simulink model "PathManager"  (R2018a)
settings: Solver=VariableStepAuto  StartTime=0.0  StopTime=10.0  RelTol=1e-3
undefined symbols (not defined in the file): check, SkywalkerX8
settings Model: Creator=David  LastModifiedBy=David

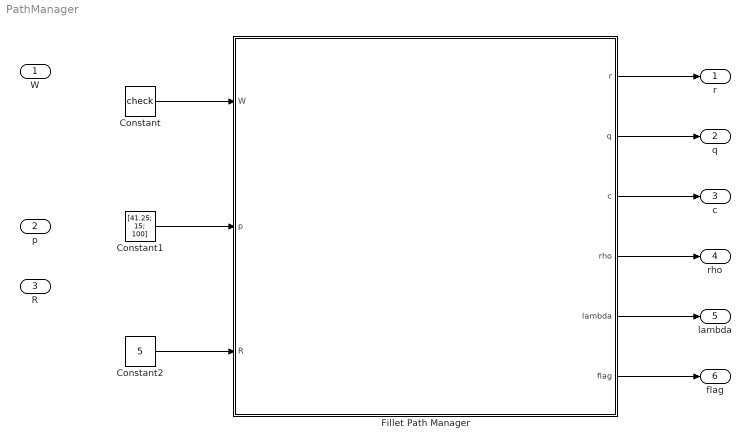
== system PathManager ==
  W : Inport
  p : Inport  Port=2
  R : Inport  Port=3
  Constant : Constant  Value=check
  Constant1 : Constant  Value=[41.25; 15; 100]
  Constant2 : Constant  Value=5
  Fillet Path Manager : Subsystem  mask{SampleTime=SkywalkerX8.GuidanceAndNavigation.SampleTime}
      mask prompts: SampleTime "Sample time (s)"
      mask DialogControl DescGroupVar Prompt: Path Manager
      mask DialogControl DescTextVar Prompt: Path manager which switches between straight line and orbit following using a fillet between waypoint transitions
      mask Display:
      | image('path_planning.png')
      | 
      | port_label('input', 1, '\bf{W} (m)', 'texMode', 'On')
      | port_label('input', 2, '\bf{p} (m)', 'texMode', 'On')
      | port_label('input', 3, 'R (m)', 'texMode', 'On')
      | 
      | port_label('output', 1, '\bf{r} (m)', 'texMode', 'On')
      | port_label('output', 2, '\bf{q} (m)', 'texMode', 'On')
      | port_label('output', 3, '\bf{c} (m)', 'texMode', 'On')
      | port_label('output', 4, '\rho (m)', 'texMode', 'On')
      | port_label('output', 5, '\lambda (m)', 'texMode', 'On')
      | port_label('output', 6, 'Flag (Unitless)', 'texMode', 'On')
  r : Outport
  q : Outport  Port=2
  c : Outport  Port=3
  rho : Outport  Port=4
  lambda : Outport  Port=5
  flag : Outport  Port=6
  wires:
  Constant/1 -> Fillet Path Manager/1(W)
  Constant1/1 -> Fillet Path Manager/2(p)
  Fillet Path Manager/1(r) -> r/1
  Fillet Path Manager/2(q) -> q/1
  Fillet Path Manager/3(c) -> c/1
  Fillet Path Manager/4(rho) -> rho/1
  Fillet Path Manager/5(lambda) -> lambda/1
  Fillet Path Manager/6(flag) -> flag/1
  Constant2/1 -> Fillet Path Manager/3(R)

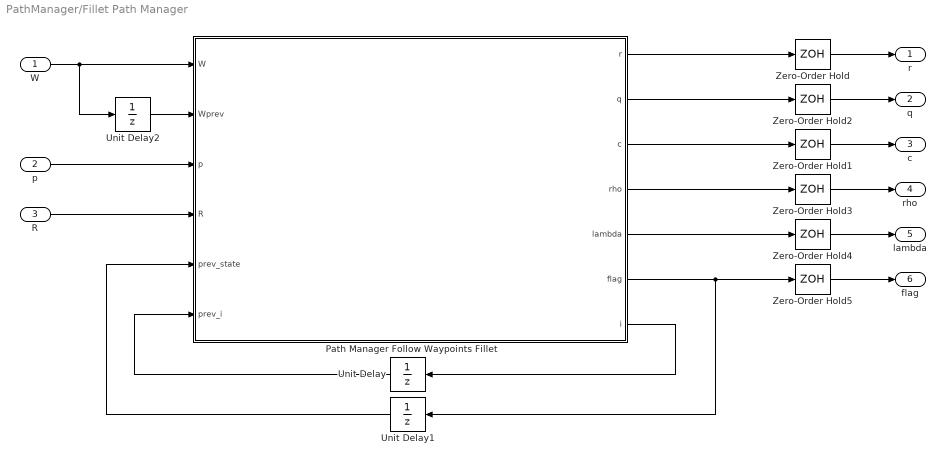
== system PathManager/Fillet Path Manager ==
  W : Inport
  p : Inport  Port=2
  R : Inport  Port=3
  Path Manager Follow Waypoints Fillet : MATLAB Function  TreatAsAtomicUnit=on
  Unit Delay : UnitDelay  InitialCondition=2  SampleTime=SampleTime
  Unit Delay1 : UnitDelay  InitialCondition=1  SampleTime=SampleTime
  Unit Delay2 : UnitDelay  SampleTime=SampleTime
  Zero-Order Hold{,1..5} (6 alike) : ZeroOrderHold  SampleTime=SampleTime
  r : Outport
  q : Outport  Port=2
  c : Outport  Port=3
  rho : Outport  Port=4
  lambda : Outport  Port=5
  flag : Outport  Port=6
  wires:
  Path Manager Follow Waypoints Fillet/2(q) -> Zero-Order Hold2/1
  Path Manager Follow Waypoints Fillet/6(flag) -> Zero-Order Hold5/1, Unit Delay1/1
  W/1 -> Unit Delay2/1, Path Manager Follow Waypoints Fillet/1(W)
  Unit Delay/1 -> Path Manager Follow Waypoints Fillet/6(prev_i)
  Path Manager Follow Waypoints Fillet/7(i) -> Unit Delay/1
  Path Manager Follow Waypoints Fillet/3(c) -> Zero-Order Hold1/1
  p/1 -> Path Manager Follow Waypoints Fillet/3(p)
  Path Manager Follow Waypoints Fillet/4(rho) -> Zero-Order Hold3/1
  Unit Delay2/1 -> Path Manager Follow Waypoints Fillet/2(Wprev)
  Path Manager Follow Waypoints Fillet/1(r) -> Zero-Order Hold/1
  Unit Delay1/1 -> Path Manager Follow Waypoints Fillet/5(prev_state)
  R/1 -> Path Manager Follow Waypoints Fillet/4(R)
  Zero-Order Hold/1 -> r/1
  Zero-Order Hold1/1 -> c/1
  Zero-Order Hold2/1 -> q/1
  Zero-Order Hold3/1 -> rho/1
  Zero-Order Hold4/1 -> lambda/1
  Zero-Order Hold5/1 -> flag/1
  Path Manager Follow Waypoints Fillet/5(lambda) -> Zero-Order Hold4/1

== matlab function PathManager/Fillet Path Manager/Path Manager Follow Waypoints Fillet ==
  data: r output size=3, 1; q output size=3, 1; c output size=3, 1; rho output size=1; lambda output size=1; W input; flag output size=1; Wprev input; p input size=3, 1; R input; prev_state input; prev_i input; i output size=1
function [r, q, c, rho, lambda, flag, i] = fcn(W, Wprev, p, R, prev_state, prev_i)
    
    [r, q, c, rho, lambda, flag, i] = pathManager_followWaypointsFillet(W, Wprev, p, R, prev_state, prev_i);

end
